simulink model "Online_Estimation_Synchrongenerator_NEW"  (R2021a)
settings: Solver=VariableStepAuto  StartTime=0.0  StopTime=10  MaxStep=0.1  MinStep=0.01  RelTol=1e-2  EnableMultiTasking=on
model workspace (MAT data in the model file):
  Ts = 0.001
settings Model: OrderedModelArguments=off  Creator=The MathWorks, Inc.  LastModifiedBy=yuganthadiyal
settings SolverCC: AlgebraicLoopSolver=TrustRegion
settings DataIOCC: LimitDataPoints=on  SaveFormat=Array  ReturnWorkspaceOutputs=off
settings OptimizationCC: LifeSpan=inf
settings DebuggingCC: SolverPrmCheckMsg=warning  SFUnexpectedBacktrackingDiag=warning  SFNoUnconditionalDefaultTransitionDiag=warning  SFExecutionAtInitializationDiag=none  SFMachineParentedDataDiag=warning  UnderSpecifiedDimensionMsg=warning  ArithmeticOperatorsInVariantConditions=warning
settings HardwareCC: ProdBitPerPointer=32  ProdBitPerSizeT=32  ProdBitPerPtrDiffT=32  ProdLargestAtomicFloat=None  ProdIntDivRoundTo=Undefined  ProdEndianess=Unspecified  ProdWordSize=32  ProdHWDeviceType=32-bit Generic
settings ModelReferenceCC: PropagateSignalLabelsOutOfModel=off
settings SFSimCC: SimUseLocalCustomCode=off  SimGenImportedTypeDefs=on  CustomCodeUndefinedFunction=UseInterfaceOnly
settings RTWCC: RTWUseLocalCustomCode=off
settings CodeAppCC: StateflowObjectComments=on
settings GRTTargetCC: TargetLangStandard=C89/C90 (ANSI)
settings ConfigComp: CovMetricSettings=dw  CovSaveCumulativeToWorkspaceVar=on  CovSaveSingleToWorkspaceVar=on  CovExternalEMLEnable=off  CovSFcnEnable=off

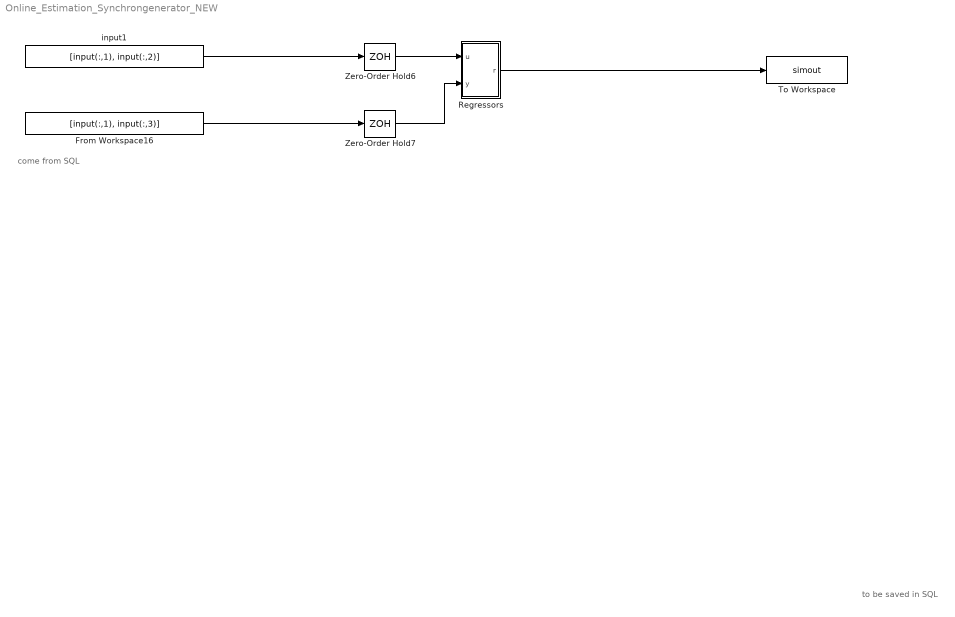
== system Online_Estimation_Synchrongenerator_NEW ==
  note: to be saved in SQL
  note: come from SQL
  From Workspace16 : FromWorkspace  VariableName=[input(:,1), input(:,3)]  SampleTime=-1
  Regressors : Subsystem
  To Workspace : ToWorkspace  VariableName=simout  SaveFormat=Timeseries  SampleTime=-1
  Zero-Order Hold6 : ZeroOrderHold  SampleTime=Ts
  Zero-Order Hold7 : ZeroOrderHold  SampleTime=Ts
  input1 : FromWorkspace  VariableName=[input(:,1), input(:,2)]  SampleTime=-1
  wires:
  From Workspace16/1 -> Zero-Order Hold7/1
  input1/1 -> Zero-Order Hold6/1
  Zero-Order Hold6/1 -> Regressors/1(u)
  Zero-Order Hold7/1 -> Regressors/2(y)
  Regressors/1(r) -> To Workspace/1

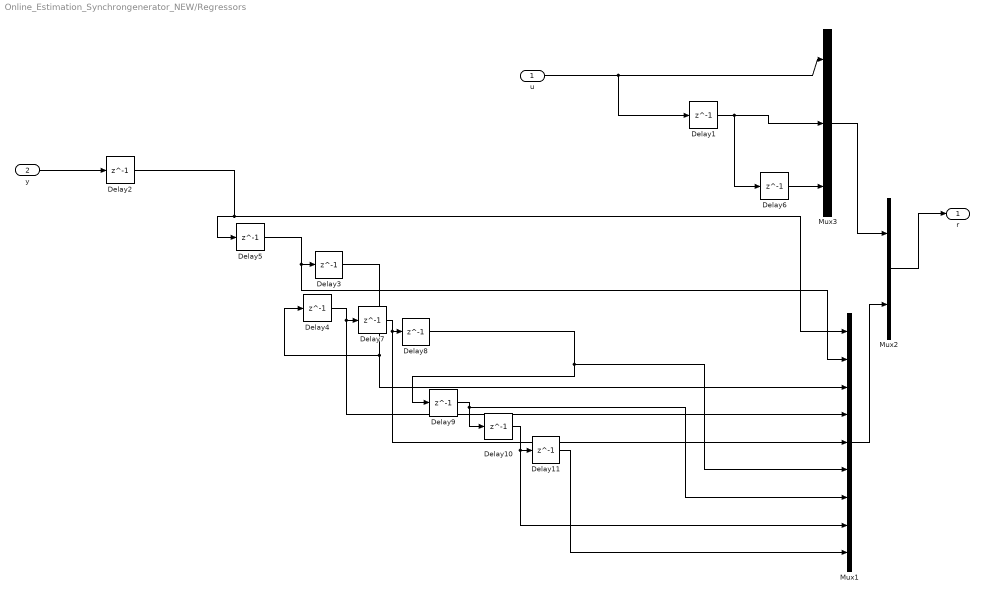
== system Online_Estimation_Synchrongenerator_NEW/Regressors ==
  u : Inport
  y : Inport  Port=2
  Delay1 : Delay  DelayLength=1  InitialCondition=1  SampleTime=Ts
  Delay{2..5,7..11} (9 alike) : Delay  DelayLength=1  InitialCondition=2  SampleTime=Ts
  Delay6 : Delay  DelayLength=1  InitialCondition=1  SampleTime=Ts
  Mux1 : Mux  Inputs=9
  Mux2 : Mux  Inputs=2
  Mux3 : Mux  Inputs=3
  r : Outport  VectorParamsAs1DForOutWhenUnconnected=off
  wires:
  Mux2/1 -> r/1
  Delay1/1 -> Delay6/1, Mux3/2
  y/1 -> Delay2/1
  Mux3/1 -> Mux2/1
  u/1 -> Delay1/1, Mux3/1
  Delay2/1 -> Delay5/1, Mux1/1
  Delay5/1 -> Delay3/1, Mux1/2
  Mux1/1 -> Mux2/2
  Delay3/1 -> Delay4/1, Mux1/3
  Delay4/1 -> Delay7/1, Mux1/4
  Delay6/1 -> Mux3/3
  Delay7/1 -> Delay8/1, Mux1/5
  Delay8/1 -> Delay9/1, Mux1/6
  Delay9/1 -> Delay10/1, Mux1/7
  Delay10/1 -> Delay11/1, Mux1/8
  Delay11/1 -> Mux1/9
